simulink model "sim06d"  (R2020a)
settings: Solver=VariableStepAuto  StartTime=0.0  StopTime=10.0  RelTol=1e-3
values from neighbouring files (symbols this model uses):
  a1 = Aw1*sqrt(2*g*(h1max-h2max))/(h1max-h2max)    [lab06.m]
  czas_skoku = 15    [lab06.m]
  du1 = 0    [lab06.m]
  du2 = 0.1*fwe1max    (= 0.5)    [lab06.m]
  h10 = fwe1/a1 + h20    [lab06.m]
  h20 = (fwe1 + fwe2)/a2    [lab06.m]
  M = [A1*A2,A1*a1+A1*a2+A2*a1,a1*a2]    [lab06.m]
  M1 = [A1,a1]    [lab06.m]
  M2 = [A2,a1+a2]    [lab06.m]
settings Model: Creator=jakub  LastModifiedBy=jakub

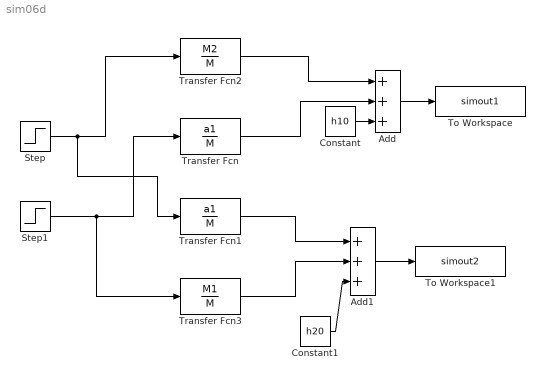
== system sim06d ==
  Add : Sum  Inputs=+++
  Add1 : Sum  Inputs=+++
  Constant : Constant  Value=h10
  Constant1 : Constant  Value=h20
  Step : Step  Time=czas_skoku  After=du1  SampleTime=0
  Step1 : Step  Time=czas_skoku  After=du2  SampleTime=0
  To Workspace : ToWorkspace  VariableName=simout1  SampleTime=-1
  To Workspace1 : ToWorkspace  VariableName=simout2  SampleTime=-1
  Transfer Fcn : TransferFcn  Numerator=a1  Denominator=M
  Transfer Fcn1 : TransferFcn  Numerator=a1  Denominator=M
  Transfer Fcn2 : TransferFcn  Numerator=M2  Denominator=M
  Transfer Fcn3 : TransferFcn  Numerator=M1  Denominator=M
  wires:
  Step/1 -> Transfer Fcn1/1, Transfer Fcn2/1
  Step1/1 -> Transfer Fcn3/1, Transfer Fcn/1
  Transfer Fcn2/1 -> Add/1
  Transfer Fcn/1 -> Add/2
  Constant/1 -> Add/3
  Add/1 -> To Workspace/1
  Transfer Fcn1/1 -> Add1/1
  Transfer Fcn3/1 -> Add1/2
  Constant1/1 -> Add1/3
  Add1/1 -> To Workspace1/1
